simulink model "Observer_for_VDP_Oscillator"  (R2022b)
settings: Solver=VariableStepAuto  StartTime=0.0  StopTime=10  RelTol=1e-3
settings Model: Creator=JianFongLee  LastModifiedBy=allen
settings DebuggingCC: UnconnectedInputMsg=warning  UnconnectedOutputMsg=warning  UnconnectedLineMsg=warning
settings ModelReferenceCC: EnableRefExpFcnMdlSchedulingChecks=on
settings RTWCC: DLArmComputeVersion=19.05

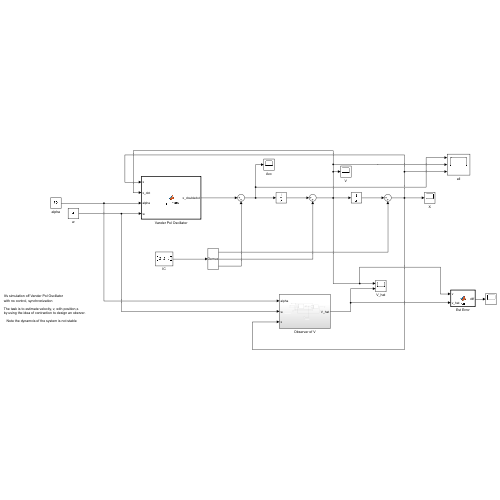
[thumbnail: Simulink's stored preview of the top-level diagram]
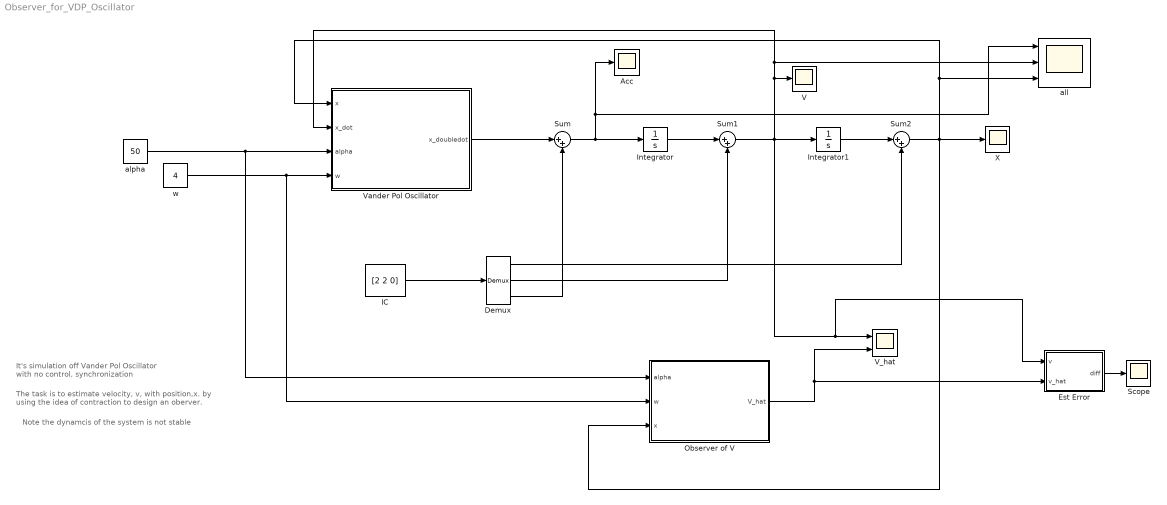
== system Observer_for_VDP_Oscillator ==
  note: Note the dynamcis of the system is not stable
  note: The task is to estimate velocity, v, with position,x.
      | by using the idea of contraction to design an oberver.
  note: It's simulation off Vander Pol Oscillator
      | with no control, synchronization
  Acc : Scope
  Demux : Demux  Outputs=3
      settings: DisplayOption=none
  Est Error : MATLAB Function  TreatAsAtomicUnit=on
  IC : Constant  Value=[2 2 0]
  Integrator : Integrator
  Integrator1 : Integrator
  Observer of V : Subsystem
  Scope : Scope
  Sum : Sum  Inputs=|++
  Sum1 : Sum  Inputs=|++
  Sum2 : Sum  Inputs=|++
  V : Scope
  V_hat : Scope  NumInputPorts=2
  Vander Pol Oscillator : MATLAB Function  TreatAsAtomicUnit=on
  X : Scope
  all : Scope  NumInputPorts=3
  alpha : Constant  Value=50
  w : Constant  Value=4
  wires:
  IC/1 -> Demux/1
  Vander Pol Oscillator/1(x_doubledot) -> Sum/1
  Demux/3 -> Sum/2
  Integrator/1 -> Sum1/1
  Demux/2 -> Sum1/2
  Integrator1/1 -> Sum2/1
  Demux/1 -> Sum2/2
  Sum2/1 -> X/1, Vander Pol Oscillator/1(x), all/3, Observer of V/3(x)
  Sum1/1 -> Est Error/1(v), V_hat/1, V/1, all/2, Vander Pol Oscillator/2(x_dot), Integrator1/1
  alpha/1 -> Observer of V/1(alpha), Vander Pol Oscillator/3(alpha)
  w/1 -> Observer of V/2(w), Vander Pol Oscillator/4(w)
  Sum/1 -> Acc/1, all/1, Integrator/1
  Observer of V/1(V_hat) -> Est Error/2(v_hat), V_hat/2
  Est Error/1(diff) -> Scope/1

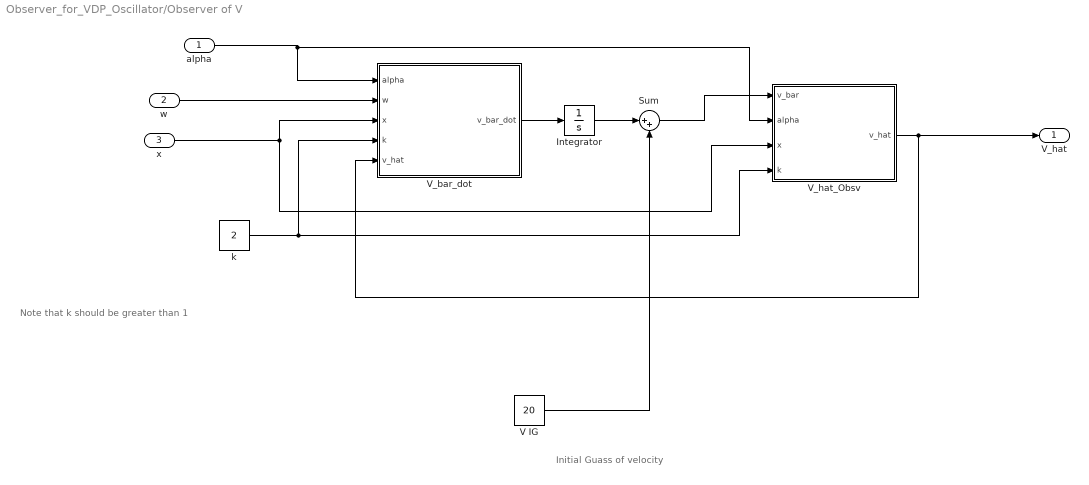
== system Observer_for_VDP_Oscillator/Observer of V ==
  note: Initial Guass of velocity
  note: Note that k should be greater than 1
  alpha : Inport
  w : Inport  Port=2
  x : Inport  Port=3
  Integrator : Integrator
  Sum : Sum  Inputs=|++
  V IG : Constant  Value=20
  V_bar_dot : MATLAB Function  TreatAsAtomicUnit=on
  V_hat_Obsv : MATLAB Function  TreatAsAtomicUnit=on
  k : Constant  Value=2
  V_hat : Outport
  wires:
  alpha/1 -> V_hat_Obsv/2(alpha), V_bar_dot/1(alpha)
  w/1 -> V_bar_dot/2(w)
  x/1 -> V_bar_dot/3(x), V_hat_Obsv/3(x)
  V_bar_dot/1(v_bar_dot) -> Integrator/1
  k/1 -> V_hat_Obsv/4(k), V_bar_dot/4(k)
  V_hat_Obsv/1(v_hat) -> V_bar_dot/5(v_hat), V_hat/1
  Integrator/1 -> Sum/1
  Sum/1 -> V_hat_Obsv/1(v_bar)
  V IG/1 -> Sum/2

== matlab function Observer_for_VDP_Oscillator/Observer of V/V_bar_dot ==
  data: alpha input; v_bar_dot output; w input; x input; k input; v_hat input
function v_bar_dot = fcn(alpha,w,x,k,v_hat)
%%% Parameters design
%%%k = 2; %%% k should be greater than 1

v_bar_dot = -alpha*(x^2+k-1)*v_hat - w^2*x;

end

== matlab function Observer_for_VDP_Oscillator/Vander Pol Oscillator ==
  data: x input; x_doubledot output; x_dot input; alpha input; w input
function x_doubledot = dynamics(x,x_dot,alpha,w)
%Parameters assignment
% alpha = 1;  %%% should be greater than 0
% w = 5;

x_doubledot = -alpha*(x^2-1)*x_dot - w^2*x;
end

%%% Dynamics of Vander Pol Oscillator
%%% x_doubledot + alpha*(x^2-1)*x_dot + w^2*x = 0;

== matlab function Observer_for_VDP_Oscillator/Observer of V/V_hat_Obsv ==
  data: v_bar input; v_hat output; alpha input; x input; k input
function v_hat = fcn(v_bar,alpha,x,k)

v_hat = v_bar + alpha*k*x;
end

== matlab function Observer_for_VDP_Oscillator/Est Error ==
  data: v input; diff output; v_hat input
function diff = fcn(v,v_hat)

diff = abs(v-v_hat);
end
